simulink model "Gs_5"  (R2015a)
settings: Solver=ode45  StartTime=0.0  StopTime=10.0  RelTol=1e-3
settings Model: Creator=Fer  LastModifiedBy=Fer

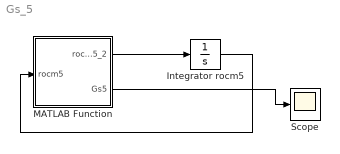
== system Gs_5 ==
  Integrator rocm5 : Integrator  InitialCondition=1.6
  MATLAB Function : MATLAB Function  TreatAsAtomicUnit=on
  Scope : Scope
  wires:
  MATLAB Function/1(rocm5_2) -> Integrator rocm5/1
  Integrator rocm5/1 -> MATLAB Function/1(rocm5)
  MATLAB Function/2(Gs5) -> Scope/1

== matlab function Gs_5/MATLAB Function ==
  data: rocm5 input; rocm5_2 output; Gs5 output
function [rocm5_2,Gs5]= Gs_5(rocm5)
%#codegen
coder.extrinsic('evalin');
vol5=1;
L=1;
s0=1;
D=1;
U=1;
roa=1;
Gs6=1;
vol5=evalin('base','vol5');
L=evalin('base','L');
s0=evalin('base','s0');
D=evalin('base','D');
U=evalin('base','U');
roa=evalin('base','roa');
Gs6=evalin('base','Gs6');
alfacm5 = acos((roa*(D+s0)-rocm5*s0)/(roa*D));
A5 = L*(s0+D*(1-cos(alfacm5)));
V5 = U*cos(alfacm5);
Gs5=3600*V5*A5*rocm5;
rocm5_2=(Gs6-Gs5)/vol5;
